simulink model "Delta_Simscape_kinematics"  (R2024b)
settings: Solver=ode15s  StartTime=0.0  StopTime=5  RelTol=1e-3
values from neighbouring files (symbols this model uses):
  s = -x*sin(phi) + y*cos(phi)    [delta.m]
undefined symbols (not defined in the file or in its folder): X, Y, Z
libraries: sm_lib x80, nesl_utility x11
(part 2 of 2)

== matlab function Delta_Simscape_kinematics/MATLAB Function1 ==
  data: x input; y input; theta1 output; z input; theta2 output; theta3 output; valid output
function [theta1, theta2, theta3, valid] = DeltaIK(x,y,z)
%#codegen
% =========================================================
% Delta机器人逆运动学
%
% 输入:
%   x,y,z       动平台中心位置 [mm]
%
% 输出:
%   theta1~3    三个主动关节角 [deg]
%   valid       1 = 有效
%               0 = 不可达
%
% 几何参数:
%   L1 = 200 mm
%   L2 = 380 mm
%   R  = 180 mm
%   r  = 80 mm
%
% 坐标定义:
%   z < 0       工作空间位于固定平台下方
%
% 角度定义:
%   theta = 0   主动臂水平向外
%   theta > 0   主动臂向下
% =========================================================


%% 机器人参数

L1 = 200.0;
L2 = 380.0;

R = 180.0;
r = 80.0;

d = R-r;


%% 三个支链方位角

phi1 = 0.0;

phi2 = 2.0*pi/3.0;

phi3 = 4.0*pi/3.0;


%% 分别计算三个关节角

[theta1,v1] = calcTheta(x,y,z,phi1,L1,L2,d);

[theta2,v2] = calcTheta(x,y,z,phi2,L1,L2,d);

[theta3,v3] = calcTheta(x,y,z,phi3,L1,L2,d);


%% 总体有效性

if (v1 > 0.5) && (v2 > 0.5) && (v3 > 0.5)

    valid = 1.0;

else

    valid = 0.0;

end

end



% =========================================================
% 单支链逆运动学
% =========================================================

function [theta,valid] = calcTheta(x,y,z,phi,L1,L2,d)

theta = 0.0;
valid = 0.0;


%% ---------------------------------------------------------
% 1. 将末端坐标转换到当前支链局部坐标
% ----------------------------------------------------------

% 径向分量
q = x*cos(phi) + y*sin(phi);

% 切向分量
s = -x*sin(phi) + y*cos(phi);


%% ---------------------------------------------------------
% 2. 固定平台与动平台铰点的径向差
% ----------------------------------------------------------

a = q-d;


%% ---------------------------------------------------------
% 3. 根据从动臂长度约束
%
% (a-L1*cos(theta))^2
% + s^2
% + (z+L1*sin(theta))^2
% = L2^2
%
% 展开得到：
%
% a*cos(theta) - z*sin(theta) = K
% ----------------------------------------------------------

K = (a*a + s*s + z*z + L1*L1 - L2*L2) ...
    /(2.0*L1);


%% ---------------------------------------------------------
% 4. 转换为标准三角方程
%
% a*cos(theta) - z*sin(theta) = K
%
% 定义：
%
% rho = sqrt(a^2+z^2)
%
% delta = atan2(-z,a)
%
% 则：
%
% rho*cos(theta-delta)=K
% ----------------------------------------------------------

rho = sqrt(a*a + z*z);

if rho < 1.0e-12
    return;
end

c = K/rho;


%% ---------------------------------------------------------
% 5. 工作空间检查
% ----------------------------------------------------------

tol = 1.0e-10;

if c > 1.0+tol
    return;
end

if c < -1.0-tol
    return;
end


% 防止浮点误差

if c > 1.0
    c = 1.0;
elseif c < -1.0
    c = -1.0;
end


%% ---------------------------------------------------------
% 6. 两个数学解
% ----------------------------------------------------------

delta = atan2(-z,a);

gamma = acos(c);


th1 = delta + gamma;

th2 = delta - gamma;


%% ---------------------------------------------------------
% 7. 归一化到 [-pi,pi]
% ----------------------------------------------------------

th1 = atan2(sin(th1),cos(th1));

th2 = atan2(sin(th2),cos(th2));


%% ---------------------------------------------------------
% 8. 选择正常Delta装配构型
%
% 当前假设机械关节范围：
%
% 0 <= theta <= 90 deg
% ----------------------------------------------------------

thetaMin = 0.0;

thetaMax = pi/2.0;


valid1 = (th1 >= thetaMin) && ...
         (th1 <= thetaMax);

valid2 = (th2 >= thetaMin) && ...
         (th2 <= thetaMax);


%% ---------------------------------------------------------
% 9. 选择物理解
% ----------------------------------------------------------

if valid1 && ~valid2

    thetaRad = th1;

elseif valid2 && ~valid1

    thetaRad = th2;

elseif valid1 && valid2

    % 两个都满足时选择较小角度
    if abs(th1) <= abs(th2)

        thetaRad = th1;

    else

        thetaRad = th2;

    end

else

    return;

end


%% ---------------------------------------------------------
% 10. 转换成 degree
% ----------------------------------------------------------

theta = thetaRad*180.0/pi;

valid = 1.0;

end
